simulink model "Practica_7"  (R2022b)
settings: Solver=VariableStepAuto  StartTime=0.0  StopTime=0.003  MaxStep=0.0000001  RelTol=1e-3
values from neighbouring files (symbols this model uses):
  C1 = 1e-7    (= 1e-07)    [Practica7.m]    (also in parametros_PRACTICA7.m)
  C2 = C1    (= 1e-07)    [Practica7.m]    (also in parametros_PRACTICA7.m)
  R1 = 1000    [Practica7.m]    (also in parametros_PRACTICA7.m)
  R2 = R1    (= 1000)    [Practica7.m]    (also in parametros_PRACTICA7.m)
  R3 = 10000    [Practica7.m]    (also in parametros_PRACTICA7.m)
  R4 = 15000    [Practica7.m]    (also in parametros_PRACTICA7.m)
settings Model: Creator=jesus  LastModifiedBy=jesus

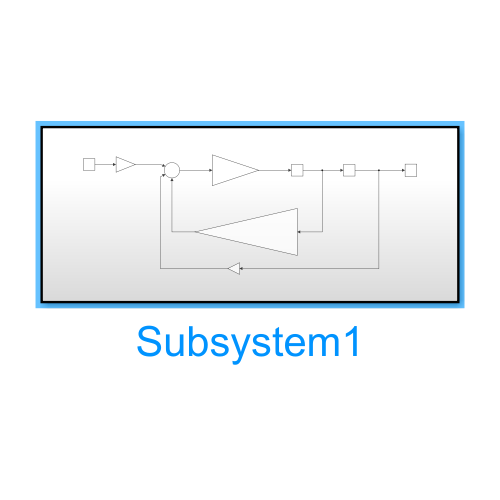
[thumbnail: Simulink's stored preview of the top-level diagram]
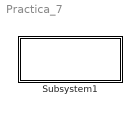
== system Practica_7 ==
  Subsystem1 : Subsystem

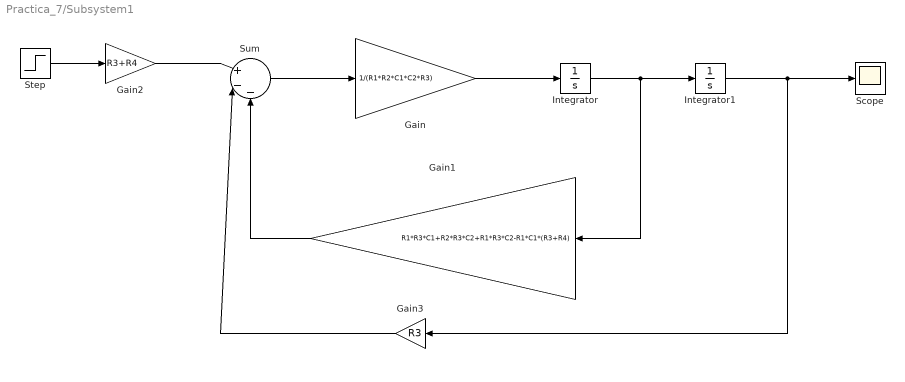
== system Practica_7/Subsystem1 ==
  Gain : Gain  Gain=1/(R1*R2*C1*C2*R3)
  Gain1 : Gain  Gain=R1*R3*C1+R2*R3*C2+R1*R3*C2-R1*C1*(R3+R4)
  Gain2 : Gain  Gain=R3+R4
  Gain3 : Gain  Gain=R3
  Integrator : Integrator
  Integrator1 : Integrator
  Scope : Scope
  Step : Step  Time=0  SampleTime=0
  Sum : Sum  Inputs=|+--
  wires:
  Integrator1/1 -> Gain3/1, Scope/1
  Sum/1 -> Gain/1
  Integrator/1 -> Gain1/1, Integrator1/1
  Gain1/1 -> Sum/3
  Gain/1 -> Integrator/1
  Gain3/1 -> Sum/2
  Step/1 -> Gain2/1
  Gain2/1 -> Sum/1
